simulink model "loopshape"  (Simulink 8.8)
settings: Solver=ode45  StartTime=0.0  StopTime=10.0  RelTol=1e-3  EnableMultiTasking=on
undefined symbols (not defined in the file): Cfd, Cs, DiscIntNeverNeededParam
libraries: simulink x1
settings Model: Creator=felipe  LastModifiedBy=mariv
settings DataIOCC: SignalLoggingSaveFormat=Dataset
settings DebuggingCC: UnderspecifiedInitializationDetection=Simplified  MergeDetectMultiDrivingBlocksExec=error  SolverPrmCheckMsg=warning  FcnCallInpInsideContextMsg=error  StateNameClashWarn=none
settings HardwareCC: TargetBitPerPointer=64  TargetBitPerSizeT=64  TargetBitPerPtrDiffT=64  TargetLongLongMode=on  TargetIntDivRoundTo=Zero  TargetEndianess=LittleEndian  TargetWordSize=64  TargetHWDeviceType=MATLAB Host  ProdEqTarget=off
settings RTWCC: SystemTargetFile=rtwsfcn.tlc  TemplateMakefile=rtwsfcn_default_tmf  Description=S-Function Target  TargetLang=C++
settings STFCustomTargetCC: ModelReferenceCompliant=off  CompOptLevelCompliant=on  MATLABClassNameForMDSCustomization=Simulink.SoftwareTarget.TargetSpecificTriggerConfigurationBase  SystemTargetFile=rtwsfcn.tlc
settings CustomProperty: Value=on

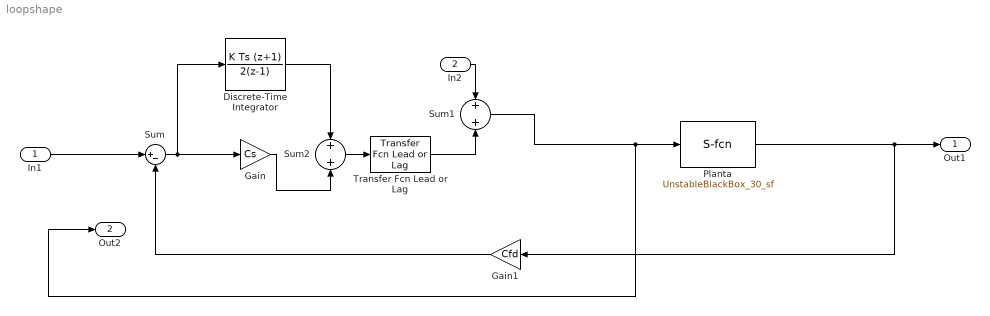
== system loopshape ==
  In1 : Inport
  In2 : Inport  Port=2
  Discrete-Time Integrator : DiscreteIntegrator  IntegratorMethod=Integration: Trapezoidal  gainval=KI  InitialConditionSetting=State (most efficient)  SampleTime=-1  ICPrevOutput=DiscIntNeverNeededParam  ICPrevScaledInput=DiscIntNeverNeededParam
  Gain : Gain  Gain=Cs
  Gain1 : Gain  Gain=Cfd
  Planta : S-Function  FunctionName=UnstableBlackBox_30_sf  SFunctionDeploymentMode=off  EnableBusSupport=off  SFcnStateName=DWORK0
      settings: SFcnIsStateOwnerBlock=on
  Sum : Sum  Inputs=|+-
  Sum1 : Sum
  Sum2 : Sum
  Transfer Fcn Lead or Lag : simulink/Discrete/Transfer Fcn Lead or Lag  PoleZ=Pz  ZeroZ=Zz  ICPrevOutput=0.0  ICPrevInput=0.0  DoSatur=off
  Out1 : Outport
  Out2 : Outport  Port=2
  wires:
  In2/1 -> Sum1/1
  Planta/1 -> Gain1/1, Out1/1
  Transfer Fcn Lead or Lag/1 -> Sum1/2
  Gain1/1 -> Sum/2
  Sum2/1 -> Transfer Fcn Lead or Lag/1
  Gain/1 -> Sum2/2
  Discrete-Time Integrator/1 -> Sum2/1
  Sum1/1 -> Out2/1, Planta/1
  Sum/1 -> Discrete-Time Integrator/1, Gain/1
  In1/1 -> Sum/1
